simulink model "Vergleich_linear_nichtlinear"  (R2021b)
settings: Solver=FixedStepAuto  StartTime=0.0  StopTime=30  FixedStep=1/1e4  RelTol=1e-3
undefined symbols (not defined in the file): A, B, C, x_Ruhe
settings Model: Creator=basti  LastModifiedBy=basti

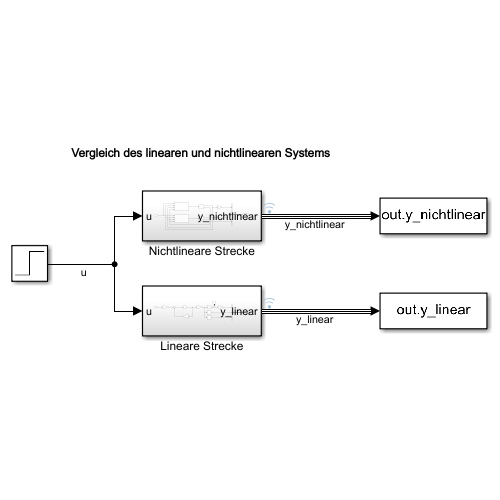
[thumbnail: Simulink's stored preview of the top-level diagram]
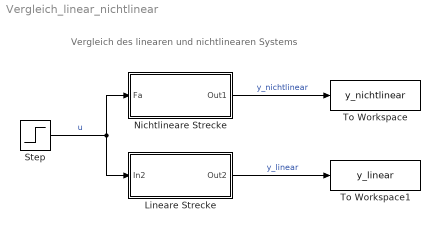
== system Vergleich_linear_nichtlinear ==
  note: Vergleich des linearen und nichtlinearen Systems
  Lineare Strecke : Subsystem
  Nichtlineare Strecke : Subsystem
  Step : Step  Time=0.5  After=30  SampleTime=0
  To Workspace : ToWorkspace  VariableName=y_nichtlinear  SaveFormat=Timeseries  SampleTime=-1
  To Workspace1 : ToWorkspace  VariableName=y_linear  SaveFormat=Timeseries  SampleTime=-1
  wires:
  Step/1 -> Nichtlineare Strecke/1(Fa), Lineare Strecke/1(In2)  "u"
  Nichtlineare Strecke/1(Out1) -> To Workspace/1  "y_nichtlinear"
  Lineare Strecke/1(Out2) -> To Workspace1/1  "y_linear"

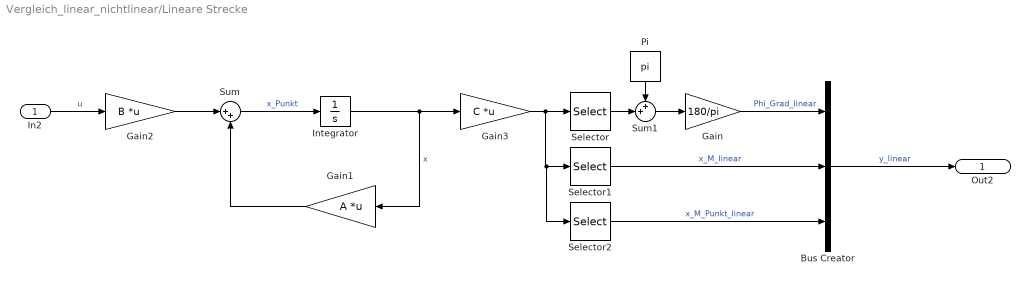
== system Vergleich_linear_nichtlinear/Lineare Strecke ==
  In2 : Inport
  Bus Creator : BusCreator  Inputs=3
  Gain : Gain  Gain=180/pi
  Gain1 : Gain  Gain=A  Multiplication=Matrix(K*u) (u vector)
  Gain2 : Gain  Gain=B  Multiplication=Matrix(K*u) (u vector)
  Gain3 : Gain  Gain=C  Multiplication=Matrix(K*u) (u vector)
  Integrator : Integrator
  Pi : Constant  Value=pi  OutDataTypeStr=Inherit: Inherit via back propagation
  Selector : Selector  InputPortWidth=3  IndexOptions=Index vector (dialog)  Indices=1  OutputSizes=1
  Selector1 : Selector  InputPortWidth=3  IndexOptions=Index vector (dialog)  Indices=2  OutputSizes=1
  Selector2 : Selector  InputPortWidth=3  IndexOptions=Index vector (dialog)  Indices=3  OutputSizes=1
  Sum : Sum  Inputs=|++
  Sum1 : Sum  Inputs=++|
  Out2 : Outport
  wires:
  In2/1 -> Gain2/1  "u"
  Gain2/1 -> Sum/1
  Gain1/1 -> Sum/2
  Sum/1 -> Integrator/1  "x_Punkt"
  Integrator/1 -> Gain3/1, Gain1/1  "x"
  Pi/1 -> Sum1/1
  Gain3/1 -> Selector2/1, Selector1/1, Selector/1
  Selector/1 -> Sum1/2
  Sum1/1 -> Gain/1
  Selector1/1 -> Bus Creator/2  "x_M_linear"
  Selector2/1 -> Bus Creator/3  "x_M_Punkt_linear"
  Gain/1 -> Bus Creator/1  "Phi_Grad_linear"
  Bus Creator/1 -> Out2/1  "y_linear"

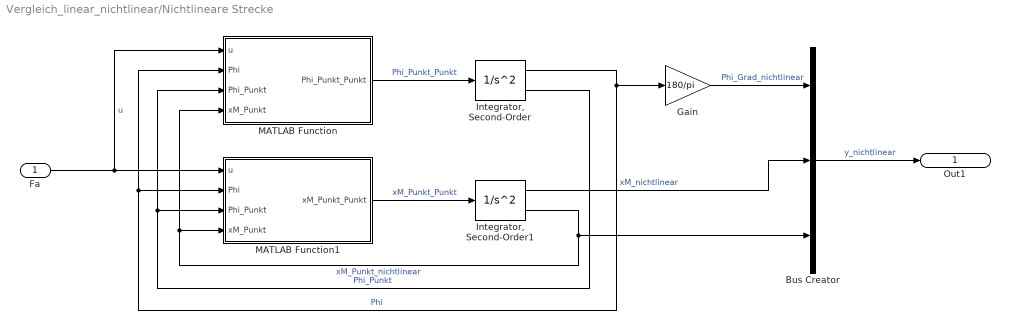
== system Vergleich_linear_nichtlinear/Nichtlineare Strecke ==
  Fa : Inport
  Bus Creator : BusCreator  Inputs=3
  Gain : Gain  Gain=180/pi
  "Integrator, Second-Order" : SecondOrderIntegrator  ICX=x_Ruhe(1, 1)  ICDXDT=x_Ruhe(2, 1)
  "Integrator, Second-Order1" : SecondOrderIntegrator  ICX=x_Ruhe(3, 1)  ICDXDT=x_Ruhe(4, 1)
  MATLAB Function : MATLAB Function  TreatAsAtomicUnit=on
  MATLAB Function1 : MATLAB Function  TreatAsAtomicUnit=on
  Out1 : Outport
  wires:
  MATLAB Function/1(Phi_Punkt_Punkt) -> "Integrator, Second-Order"/1  "Phi_Punkt_Punkt"
  MATLAB Function1/1(xM_Punkt_Punkt) -> "Integrator, Second-Order1"/1  "xM_Punkt_Punkt"
  "Integrator, Second-Order1"/2 -> Bus Creator/3, MATLAB Function1/4(xM_Punkt), MATLAB Function/4(xM_Punkt)  "xM_Punkt_nichtlinear"
  "Integrator, Second-Order"/2 -> MATLAB Function/3(Phi_Punkt), MATLAB Function1/3(Phi_Punkt)  "Phi_Punkt"
  "Integrator, Second-Order"/1 -> MATLAB Function/2(Phi), MATLAB Function1/2(Phi), Gain/1  "Phi"
  Fa/1 -> MATLAB Function/1(u), MATLAB Function1/1(u)  "u"
  Gain/1 -> Bus Creator/1  "Phi_Grad_nichtlinear"
  "Integrator, Second-Order1"/1 -> Bus Creator/2  "xM_nichtlinear"
  Bus Creator/1 -> Out1/1  "y_nichtlinear"

== matlab function Vergleich_linear_nichtlinear/Nichtlineare Strecke/MATLAB Function1 ==
  data: u input; xM_Punkt_Punkt output; Phi input; Phi_Punkt input; xM_Punkt input
function xM_Punkt_Punkt = fcn(u, Phi, Phi_Punkt, xM_Punkt)
    % Konstanten
    c = Konstanten();

    % Berechnung
    xM_Punkt_Punkt = (c.g*tan(Phi)+1/(c.m*cos(Phi)^2)*(c.d*xM_Punkt-u)-(c.l*Phi_Punkt^2*tan(Phi))/cos(Phi)-(c.d_Mf*Phi_Punkt)/(c.m*c.l*cos(Phi)))/(1-(c.M+c.m)/(c.m*cos(Phi)^2));

== matlab function Vergleich_linear_nichtlinear/Nichtlineare Strecke/MATLAB Function ==
  data: u input; Phi_Punkt_Punkt output; Phi input; Phi_Punkt input; xM_Punkt input
function Phi_Punkt_Punkt = fcn(u, Phi, Phi_Punkt, xM_Punkt)
    % Konstanten
    c = Konstanten();

    % Berechnung
    Phi_Punkt_Punkt = ((u-c.g*tan(Phi)*(c.M+c.m)-c.d*xM_Punkt)/(c.m*c.l*cos(Phi))+c.d_Mf*Phi_Punkt*(c.M/(c.m^2*c.l^2*cos(Phi)^2)+1/(c.m*c.l^2*cos(Phi)^2))+Phi_Punkt^2*tan(Phi))/(1-(1/cos(Phi)^2)-c.M/(c.m*cos(Phi)^2));
